simulink model "cuurent_controlled_circuit"  (R2022a)
settings: Solver=VariableStepAuto  StartTime=0.0  StopTime=25.0  RelTol=1e-3
undefined symbols (not defined in the file or in its folder): DiscIntNeverNeededParam
libraries: fl_lib x82, nesl_utility x65, eeRmsMeasurement x34, eePowerMeasurement x17, ee_lib x16
(part 2 of 3)

== system cuurent_controlled_circuit/Subsystem2 ==
  Display3 : Display
  Display4 : Display
  Display5 : Display
  PS-Simulink Converter2 : nesl_utility/PS-Simulink Converter  PhysicalDomain=network_engine_domain  SubClassName=ps_output  LeftPortType=input  RightPortType=output  PseudoPeriodic=off  Frequencies=[]  VectorFormat=inherit  Unit=inherit  AffineConversion=off
      settings: SourceProductBaseCode=SS,PW,VE
  PS-Simulink Converter3 : nesl_utility/PS-Simulink Converter  PhysicalDomain=network_engine_domain  SubClassName=ps_output  LeftPortType=input  RightPortType=output  PseudoPeriodic=off  Frequencies=[]  VectorFormat=inherit  Unit=inherit  AffineConversion=off
      settings: SourceProductBaseCode=SS,PW,VE
  Power Measurement2 : eePowerMeasurement/Power Measurement  LabelModeActiveChoice=Continuous  F=50  K=[0 1 2 3]  Ts=0
      settings: SourceProductBaseCode=PS
  RMS Measurement2 : eeRmsMeasurement/RMS Measurement  LabelModeActiveChoice=Total  F=50  SpecifyHarmonics=off  K=[0 1 2]  Ts=0
      settings: SourceProductBaseCode=PS
  RMS Measurement3 : eeRmsMeasurement/RMS Measurement  LabelModeActiveChoice=Total  F=50  SpecifyHarmonics=off  K=[0 1 2]  Ts=0
      settings: SourceProductBaseCode=PS
  Scope{6..10} (5 alike) : Scope
  input : PMIOPort  Side=Left
  input1 : PMIOPort  Port=2  Side=Left
  Q : Outport
  wires:
  Power Measurement2/2 -> Q/1
  PS-Simulink Converter3/1 -> RMS Measurement3/1, Scope8/1
  Power Measurement2/1 -> Display5/1, Scope10/1
  RMS Measurement2/1 -> Scope7/1, Display3/1, Power Measurement2/1
  PS-Simulink Converter2/1 -> RMS Measurement2/1, Scope6/1
  RMS Measurement3/1 -> Power Measurement2/2, Scope9/1, Display4/1
  connections:
  PS-Simulink Converter3/LConn1 -- input1/RConn1
  PS-Simulink Converter2/LConn1 -- input/RConn1

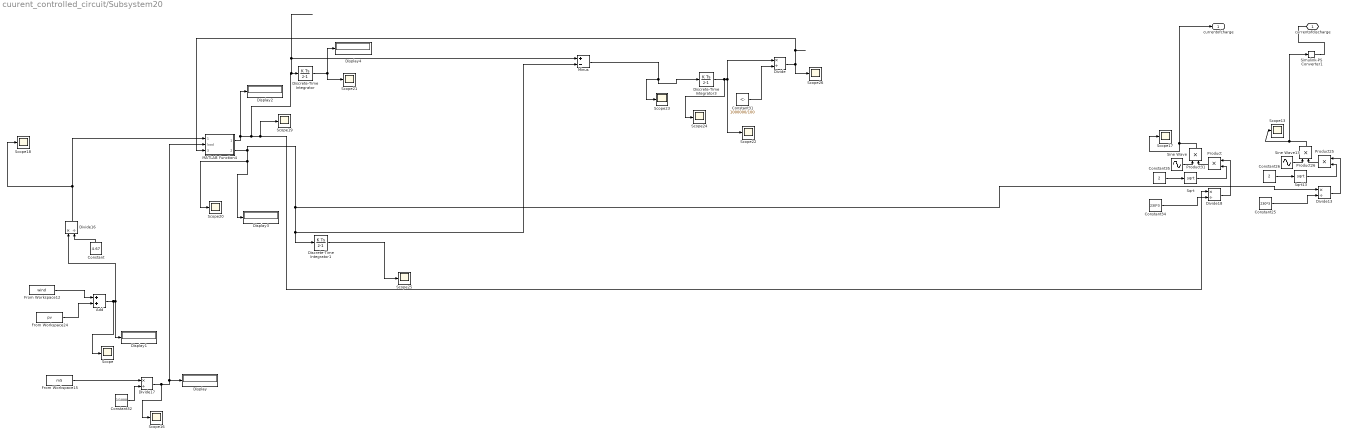
== system cuurent_controlled_circuit/Subsystem20 ==
  Add : Sum
  Constant : Constant  Value=4.67
  Constant25 : Constant  Value=230*3
  Constant26 : Constant  Value=2
  Constant31 : Constant  Value=1000000/100
  Constant32 : Constant  Value=1/1000
  Constant34 : Constant  Value=230*3
  Constant35 : Constant  Value=2
  Discrete-Time Integrator : DiscreteIntegrator  ICPrevOutput=DiscIntNeverNeededParam  ICPrevScaledInput=DiscIntNeverNeededParam
  Discrete-Time Integrator1 : DiscreteIntegrator  ICPrevOutput=DiscIntNeverNeededParam  ICPrevScaledInput=DiscIntNeverNeededParam
  Discrete-Time Integrator3 : DiscreteIntegrator  InitialCondition=500000  ICPrevOutput=DiscIntNeverNeededParam  ICPrevScaledInput=DiscIntNeverNeededParam
  Display{,1..4} (5 alike) : Display
  Divide{,13,16..18} (5 alike) : Product  Inputs=*/
  From Workspace12 : FromWorkspace  VariableName=wind  SampleTime=1  Interpolate=off  OutputAfterFinalValue=Holding final value
  From Workspace15 : FromWorkspace  VariableName=m5  SampleTime=1  Interpolate=off  OutputAfterFinalValue=Holding final value
  From Workspace24 : FromWorkspace  VariableName=pv  SampleTime=1  Interpolate=off  OutputAfterFinalValue=Holding final value
  MATLAB Function4 : MATLAB Function  TreatAsAtomicUnit=on
  Minus : Sum  Inputs=+-
  Product{,25..26,31} (4 alike) : Product
  Scope{,13,16..26} (13 alike) : Scope
  Simulink-PS Converter1 : nesl_utility/Simulink-PS Converter  PhysicalDomain=network_engine_domain  SubClassName=ps_input  LeftPortType=input  RightPortType=output  PseudoPeriodic=off  Frequencies=[]  NoiseDistribution=none  NoiseParameters=[]  Unit=1  AffineConversion=off  FilteringAndDerivatives=provide  SimscapeFilterOrder=1  InputFilterTimeConstant=0.001  UdotUserProvided=0
      settings: SourceProductBaseCode=SS,PW,VE
  Sine Wave : Sin  TimeSource=Use external signal  Frequency=314.6  Phase=240  SampleTime=0
  Sine Wave13 : Sin  Frequency=314.6  Phase=240  SampleTime=0
  Sqrt : Sqrt
  Sqrt13 : Sqrt
  currentofdischarge : PMIOPort  Side=Right
  currentofcharge : Outport
  wires:
  MATLAB Function4/1(charge) -> Minus/1, Discrete-Time Integrator/1, Divide18/1, Scope19/1, Display2/1
  MATLAB Function4/2(discharge) -> Divide13/1, Minus/2, Discrete-Time Integrator1/1, Scope20/1, Display3/1
  Divide/1 -> MATLAB Function4/3(batterycharge), Scope26/1
  Sine Wave13/1 -> Product26/1
  Product26/1 -> Simulink-PS Converter1/1, Scope13/1
  Discrete-Time Integrator/1 -> Display4/1, Scope21/1
  From Workspace24/1 -> Add/2
  Constant35/1 -> Sqrt/1
  Constant26/1 -> Sqrt13/1
  Product31/1 -> currentofcharge/1, Scope17/1
  Divide17/1 -> Scope16/1, MATLAB Function4/2(load), Display/1
  Divide13/1 -> Product25/1
  Add/1 -> Scope/1, Divide16/1, Display1/1
  Constant31/1 -> Divide/2
  Discrete-Time Integrator1/1 -> Scope25/1
  From Workspace15/1 -> Divide17/1
  Constant32/1 -> Divide17/2
  Minus/1 -> Discrete-Time Integrator3/1, Scope23/1
  Divide18/1 -> Product/1
  Discrete-Time Integrator3/1 -> Scope24/1, Divide/1, Scope22/1
  Product/1 -> Product31/2
  Product25/1 -> Product26/2
  Constant25/1 -> Divide13/2
  Constant/1 -> Divide16/2
  Divide16/1 -> Scope18/1, MATLAB Function4/1(pvandwind)
  Sine Wave/1 -> Product31/1
  Constant34/1 -> Divide18/2
  Sqrt/1 -> Product/2
  Sqrt13/1 -> Product25/2
  From Workspace12/1 -> Add/1
  connections:
  Simulink-PS Converter1/RConn1 -- currentofdischarge/RConn1

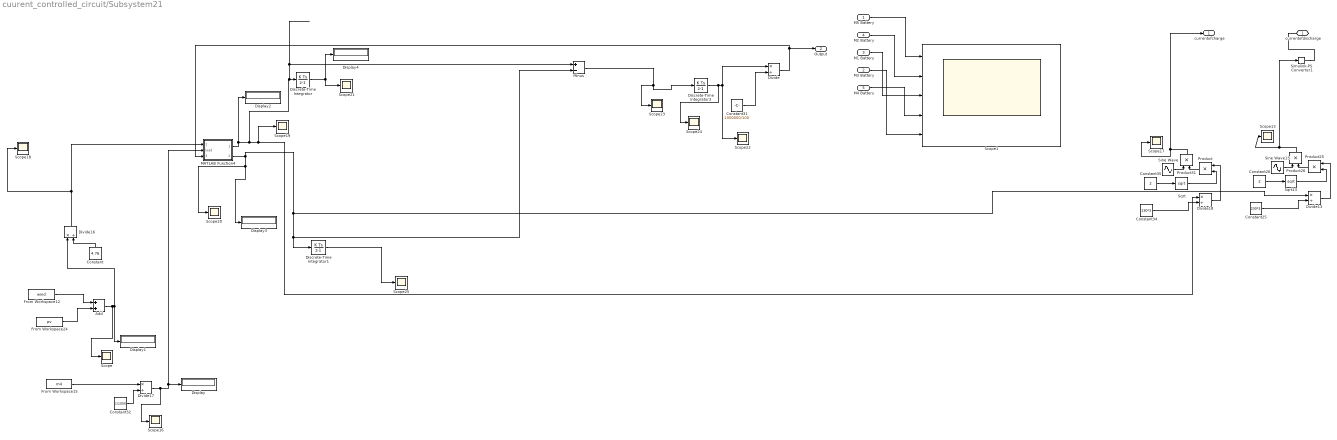
== system cuurent_controlled_circuit/Subsystem21 ==
  M5 Battery : Inport
  M3 Battery : Inport  Port=2
  M1 Battery : Inport  Port=3
  M2 Battery : Inport  Port=4
  M4 Battery : Inport  Port=5
  Add : Sum
  Constant : Constant  Value=4.76
  Constant25 : Constant  Value=230*3
  Constant26 : Constant  Value=2
  Constant31 : Constant  Value=1000000/100
  Constant32 : Constant  Value=1/1000
  Constant34 : Constant  Value=230*3
  Constant35 : Constant  Value=2
  Discrete-Time Integrator : DiscreteIntegrator  ICPrevOutput=DiscIntNeverNeededParam  ICPrevScaledInput=DiscIntNeverNeededParam
  Discrete-Time Integrator1 : DiscreteIntegrator  ICPrevOutput=DiscIntNeverNeededParam  ICPrevScaledInput=DiscIntNeverNeededParam
  Discrete-Time Integrator3 : DiscreteIntegrator  InitialCondition=500000  ICPrevOutput=DiscIntNeverNeededParam  ICPrevScaledInput=DiscIntNeverNeededParam
  Display{,1..4} (5 alike) : Display
  Divide{,13,16..18} (5 alike) : Product  Inputs=*/
  From Workspace12 : FromWorkspace  VariableName=wind  SampleTime=1  Interpolate=off  OutputAfterFinalValue=Holding final value
  From Workspace15 : FromWorkspace  VariableName=m4  SampleTime=1  Interpolate=off  OutputAfterFinalValue=Holding final value
  From Workspace24 : FromWorkspace  VariableName=pv  SampleTime=1  Interpolate=off  OutputAfterFinalValue=Holding final value
  MATLAB Function4 : MATLAB Function  TreatAsAtomicUnit=on
  Minus : Sum  Inputs=+-
  Product{,25..26,31} (4 alike) : Product
  Scope{,13,16..25} (12 alike) : Scope
  Scope1 : Scope  NumInputPorts=5
  Simulink-PS Converter1 : nesl_utility/Simulink-PS Converter  PhysicalDomain=network_engine_domain  SubClassName=ps_input  LeftPortType=input  RightPortType=output  PseudoPeriodic=off  Frequencies=[]  NoiseDistribution=none  NoiseParameters=[]  Unit=1  AffineConversion=off  FilteringAndDerivatives=provide  SimscapeFilterOrder=1  InputFilterTimeConstant=0.001  UdotUserProvided=0
      settings: SourceProductBaseCode=SS,PW,VE
  Sine Wave : Sin  Frequency=314.6  SampleTime=0
  Sine Wave13 : Sin  Frequency=314.6  SampleTime=0
  Sqrt : Sqrt
  Sqrt13 : Sqrt
  currentofdischarge : PMIOPort  Side=Right
  currentofcharge : Outport
  Output : Outport  Port=2
  wires:
  MATLAB Function4/1(charge) -> Minus/1, Discrete-Time Integrator/1, Divide18/1, Scope19/1, Display2/1
  MATLAB Function4/2(discharge) -> Divide13/1, Minus/2, Discrete-Time Integrator1/1, Scope20/1, Display3/1
  Sine Wave13/1 -> Product26/1
  Product26/1 -> Simulink-PS Converter1/1, Scope13/1
  Discrete-Time Integrator/1 -> Display4/1, Scope21/1
  From Workspace24/1 -> Add/2
  Constant35/1 -> Sqrt/1
  Constant26/1 -> Sqrt13/1
  Product31/1 -> currentofcharge/1, Scope17/1
  Divide17/1 -> Scope16/1, MATLAB Function4/2(load), Display/1
  Divide13/1 -> Product25/1
  Add/1 -> Scope/1, Divide16/1, Display1/1
  Constant31/1 -> Divide/2
  Discrete-Time Integrator1/1 -> Scope25/1
  From Workspace15/1 -> Divide17/1
  Constant32/1 -> Divide17/2
  Minus/1 -> Discrete-Time Integrator3/1, Scope23/1
  Divide18/1 -> Product/1
  Discrete-Time Integrator3/1 -> Scope24/1, Divide/1, Scope22/1
  Product/1 -> Product31/2
  Product25/1 -> Product26/2
  Constant25/1 -> Divide13/2
  Constant/1 -> Divide16/2
  Divide16/1 -> Scope18/1, MATLAB Function4/1(pvandwind)
  Sine Wave/1 -> Product31/1
  Constant34/1 -> Divide18/2
  Sqrt/1 -> Product/2
  Sqrt13/1 -> Product25/2
  From Workspace12/1 -> Add/1
  M5 Battery/1 -> Scope1/1
  M2 Battery/1 -> Scope1/2
  M1 Battery/1 -> Scope1/3
  M3 Battery/1 -> Scope1/5
  Divide/1 -> Output/1, MATLAB Function4/3(batterycharge)
  M4 Battery/1 -> Scope1/4
  connections:
  Simulink-PS Converter1/RConn1 -- currentofdischarge/RConn1

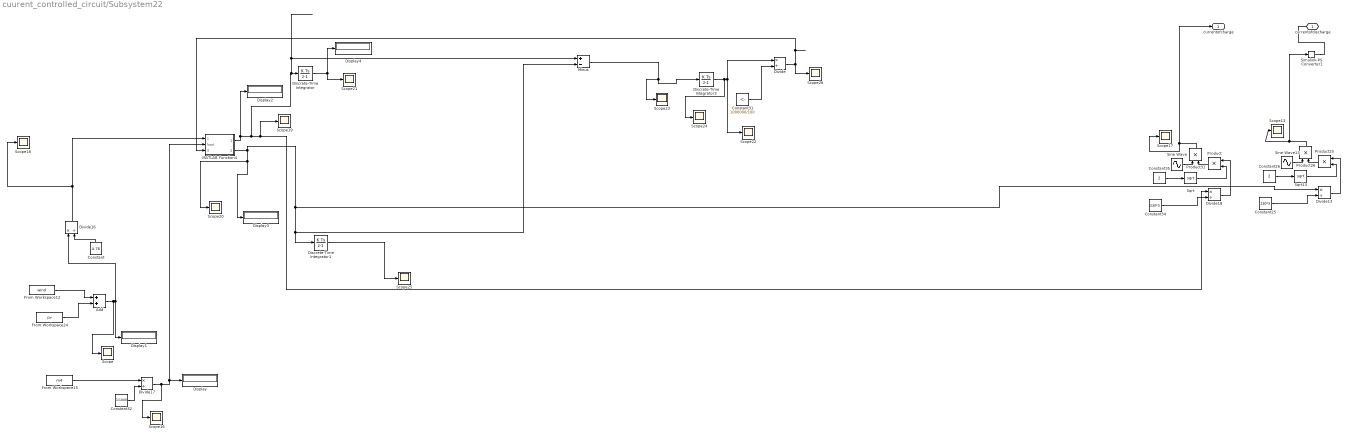
== system cuurent_controlled_circuit/Subsystem22 ==
  Add : Sum
  Constant : Constant  Value=4.76
  Constant25 : Constant  Value=230*3
  Constant26 : Constant  Value=2
  Constant31 : Constant  Value=1000000/100
  Constant32 : Constant  Value=1/1000
  Constant34 : Constant  Value=230*3
  Constant35 : Constant  Value=2
  Discrete-Time Integrator : DiscreteIntegrator  ICPrevOutput=DiscIntNeverNeededParam  ICPrevScaledInput=DiscIntNeverNeededParam
  Discrete-Time Integrator1 : DiscreteIntegrator  ICPrevOutput=DiscIntNeverNeededParam  ICPrevScaledInput=DiscIntNeverNeededParam
  Discrete-Time Integrator3 : DiscreteIntegrator  InitialCondition=500000  ICPrevOutput=DiscIntNeverNeededParam  ICPrevScaledInput=DiscIntNeverNeededParam
  Display{,1..4} (5 alike) : Display
  Divide{,13,16..18} (5 alike) : Product  Inputs=*/
  From Workspace12 : FromWorkspace  VariableName=wind  SampleTime=1  Interpolate=off  OutputAfterFinalValue=Holding final value
  From Workspace15 : FromWorkspace  VariableName=m4  SampleTime=1  Interpolate=off  OutputAfterFinalValue=Holding final value
  From Workspace24 : FromWorkspace  VariableName=pv  SampleTime=1  Interpolate=off  OutputAfterFinalValue=Holding final value
  MATLAB Function4 : MATLAB Function  TreatAsAtomicUnit=on
  Minus : Sum  Inputs=+-
  Product{,25..26,31} (4 alike) : Product
  Scope{,13,16..26} (13 alike) : Scope
  Simulink-PS Converter1 : nesl_utility/Simulink-PS Converter  PhysicalDomain=network_engine_domain  SubClassName=ps_input  LeftPortType=input  RightPortType=output  PseudoPeriodic=off  Frequencies=[]  NoiseDistribution=none  NoiseParameters=[]  Unit=1  AffineConversion=off  FilteringAndDerivatives=provide  SimscapeFilterOrder=1  InputFilterTimeConstant=0.001  UdotUserProvided=0
      settings: SourceProductBaseCode=SS,PW,VE
  Sine Wave : Sin  Frequency=314.6  Phase=120  SampleTime=0
  Sine Wave13 : Sin  Frequency=314.6  Phase=120  SampleTime=0
  Sqrt : Sqrt
  Sqrt13 : Sqrt
  currentofdischarge : PMIOPort  Side=Right
  currentofcharge : Outport
  wires:
  MATLAB Function4/1(charge) -> Minus/1, Discrete-Time Integrator/1, Divide18/1, Scope19/1, Display2/1
  MATLAB Function4/2(discharge) -> Divide13/1, Minus/2, Discrete-Time Integrator1/1, Scope20/1, Display3/1
  Divide/1 -> MATLAB Function4/3(batterycharge), Scope26/1
  Sine Wave13/1 -> Product26/1
  Product26/1 -> Simulink-PS Converter1/1, Scope13/1
  Discrete-Time Integrator/1 -> Display4/1, Scope21/1
  From Workspace24/1 -> Add/2
  Constant35/1 -> Sqrt/1
  Constant26/1 -> Sqrt13/1
  Product31/1 -> currentofcharge/1, Scope17/1
  Divide17/1 -> Scope16/1, MATLAB Function4/2(load), Display/1
  Divide13/1 -> Product25/1
  Add/1 -> Scope/1, Divide16/1, Display1/1
  Constant31/1 -> Divide/2
  Discrete-Time Integrator1/1 -> Scope25/1
  From Workspace15/1 -> Divide17/1
  Constant32/1 -> Divide17/2
  Minus/1 -> Discrete-Time Integrator3/1, Scope23/1
  Divide18/1 -> Product/1
  Discrete-Time Integrator3/1 -> Scope24/1, Divide/1, Scope22/1
  Product/1 -> Product31/2
  Product25/1 -> Product26/2
  Constant25/1 -> Divide13/2
  Constant/1 -> Divide16/2
  Divide16/1 -> Scope18/1, MATLAB Function4/1(pvandwind)
  Sine Wave/1 -> Product31/1
  Constant34/1 -> Divide18/2
  Sqrt/1 -> Product/2
  Sqrt13/1 -> Product25/2
  From Workspace12/1 -> Add/1
  connections:
  Simulink-PS Converter1/RConn1 -- currentofdischarge/RConn1

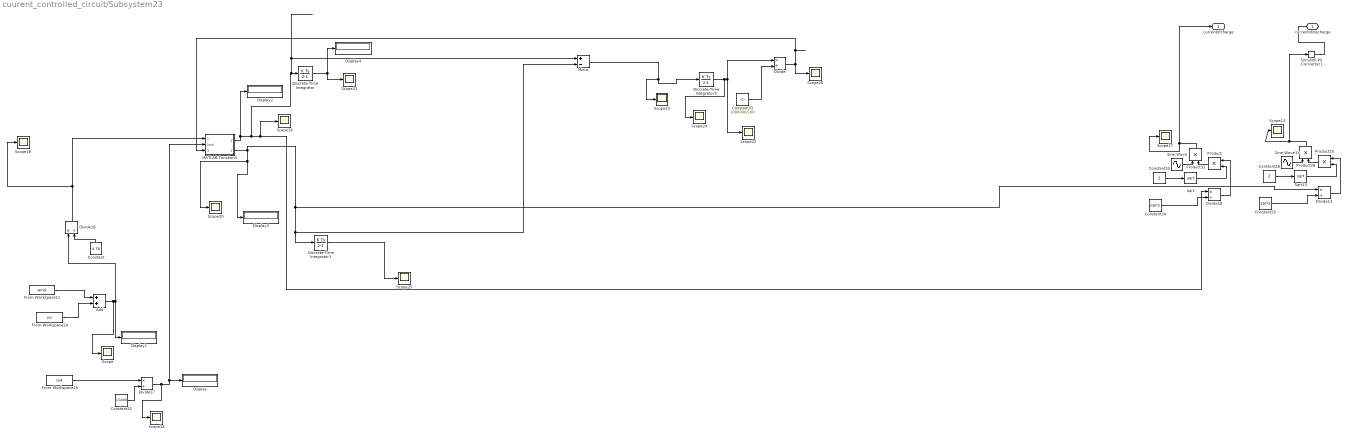
== system cuurent_controlled_circuit/Subsystem23 ==
  Add : Sum
  Constant : Constant  Value=4.76
  Constant25 : Constant  Value=230*3
  Constant26 : Constant  Value=2
  Constant31 : Constant  Value=1000000/100
  Constant32 : Constant  Value=1/1000
  Constant34 : Constant  Value=230*3
  Constant35 : Constant  Value=2
  Discrete-Time Integrator : DiscreteIntegrator  ICPrevOutput=DiscIntNeverNeededParam  ICPrevScaledInput=DiscIntNeverNeededParam
  Discrete-Time Integrator1 : DiscreteIntegrator  ICPrevOutput=DiscIntNeverNeededParam  ICPrevScaledInput=DiscIntNeverNeededParam
  Discrete-Time Integrator3 : DiscreteIntegrator  InitialCondition=500000  ICPrevOutput=DiscIntNeverNeededParam  ICPrevScaledInput=DiscIntNeverNeededParam
  Display{,1..4} (5 alike) : Display
  Divide{,13,16..18} (5 alike) : Product  Inputs=*/
  From Workspace12 : FromWorkspace  VariableName=wind  SampleTime=1  Interpolate=off  OutputAfterFinalValue=Holding final value
  From Workspace15 : FromWorkspace  VariableName=m4  SampleTime=1  Interpolate=off  OutputAfterFinalValue=Holding final value
  From Workspace24 : FromWorkspace  VariableName=pv  SampleTime=1  Interpolate=off  OutputAfterFinalValue=Holding final value
  MATLAB Function4 : MATLAB Function  TreatAsAtomicUnit=on
  Minus : Sum  Inputs=+-
  Product{,25..26,31} (4 alike) : Product
  Scope{,13,16..26} (13 alike) : Scope
  Simulink-PS Converter1 : nesl_utility/Simulink-PS Converter  PhysicalDomain=network_engine_domain  SubClassName=ps_input  LeftPortType=input  RightPortType=output  PseudoPeriodic=off  Frequencies=[]  NoiseDistribution=none  NoiseParameters=[]  Unit=1  AffineConversion=off  FilteringAndDerivatives=provide  SimscapeFilterOrder=1  InputFilterTimeConstant=0.001  UdotUserProvided=0
      settings: SourceProductBaseCode=SS,PW,VE
  Sine Wave : Sin  Frequency=314.6  Phase=240  SampleTime=0
  Sine Wave13 : Sin  Frequency=314.6  Phase=240  SampleTime=0
  Sqrt : Sqrt
  Sqrt13 : Sqrt
  currentofdischarge : PMIOPort  Side=Right
  currentofcharge : Outport
  wires:
  MATLAB Function4/1(charge) -> Minus/1, Discrete-Time Integrator/1, Divide18/1, Scope19/1, Display2/1
  MATLAB Function4/2(discharge) -> Divide13/1, Minus/2, Discrete-Time Integrator1/1, Scope20/1, Display3/1
  Divide/1 -> MATLAB Function4/3(batterycharge), Scope26/1
  Sine Wave13/1 -> Product26/1
  Product26/1 -> Simulink-PS Converter1/1, Scope13/1
  Discrete-Time Integrator/1 -> Display4/1, Scope21/1
  From Workspace24/1 -> Add/2
  Constant35/1 -> Sqrt/1
  Constant26/1 -> Sqrt13/1
  Product31/1 -> currentofcharge/1, Scope17/1
  Divide17/1 -> Scope16/1, MATLAB Function4/2(load), Display/1
  Divide13/1 -> Product25/1
  Add/1 -> Scope/1, Divide16/1, Display1/1
  Constant31/1 -> Divide/2
  Discrete-Time Integrator1/1 -> Scope25/1
  From Workspace15/1 -> Divide17/1
  Constant32/1 -> Divide17/2
  Minus/1 -> Discrete-Time Integrator3/1, Scope23/1
  Divide18/1 -> Product/1
  Discrete-Time Integrator3/1 -> Scope24/1, Divide/1, Scope22/1
  Product/1 -> Product31/2
  Product25/1 -> Product26/2
  Constant25/1 -> Divide13/2
  Constant/1 -> Divide16/2
  Divide16/1 -> Scope18/1, MATLAB Function4/1(pvandwind)
  Sine Wave/1 -> Product31/1
  Constant34/1 -> Divide18/2
  Sqrt/1 -> Product/2
  Sqrt13/1 -> Product25/2
  From Workspace12/1 -> Add/1
  connections:
  Simulink-PS Converter1/RConn1 -- currentofdischarge/RConn1

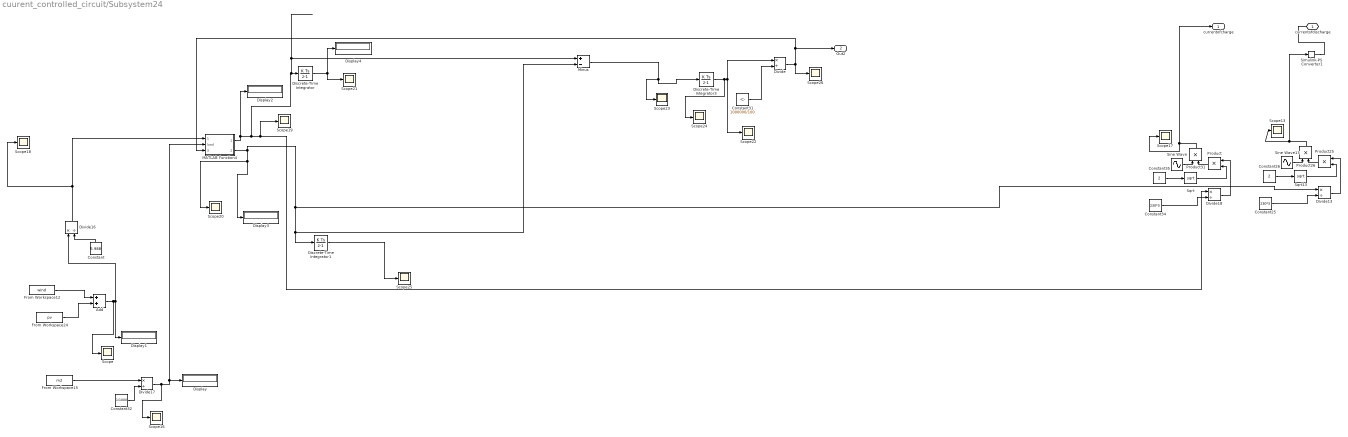
== system cuurent_controlled_circuit/Subsystem24 ==
  Add : Sum
  Constant : Constant  Value=5.988
  Constant25 : Constant  Value=230*3
  Constant26 : Constant  Value=2
  Constant31 : Constant  Value=1000000/100
  Constant32 : Constant  Value=1/1000
  Constant34 : Constant  Value=230*3
  Constant35 : Constant  Value=2
  Discrete-Time Integrator : DiscreteIntegrator  ICPrevOutput=DiscIntNeverNeededParam  ICPrevScaledInput=DiscIntNeverNeededParam
  Discrete-Time Integrator1 : DiscreteIntegrator  ICPrevOutput=DiscIntNeverNeededParam  ICPrevScaledInput=DiscIntNeverNeededParam
  Discrete-Time Integrator3 : DiscreteIntegrator  InitialCondition=500000  ICPrevOutput=DiscIntNeverNeededParam  ICPrevScaledInput=DiscIntNeverNeededParam
  Display{,1..4} (5 alike) : Display
  Divide{,13,16..18} (5 alike) : Product  Inputs=*/
  From Workspace12 : FromWorkspace  VariableName=wind  SampleTime=1  Interpolate=off  OutputAfterFinalValue=Holding final value
  From Workspace15 : FromWorkspace  VariableName=m2  SampleTime=1  Interpolate=off  OutputAfterFinalValue=Holding final value
  From Workspace24 : FromWorkspace  VariableName=pv  SampleTime=1  Interpolate=off  OutputAfterFinalValue=Holding final value
  MATLAB Function4 : MATLAB Function  TreatAsAtomicUnit=on
  Minus : Sum  Inputs=+-
  Product{,25..26,31} (4 alike) : Product
  Scope{,13,16..26} (13 alike) : Scope
  Simulink-PS Converter1 : nesl_utility/Simulink-PS Converter  PhysicalDomain=network_engine_domain  SubClassName=ps_input  LeftPortType=input  RightPortType=output  PseudoPeriodic=off  Frequencies=[]  NoiseDistribution=none  NoiseParameters=[]  Unit=1  AffineConversion=off  FilteringAndDerivatives=provide  SimscapeFilterOrder=1  InputFilterTimeConstant=0.001  UdotUserProvided=0
      settings: SourceProductBaseCode=SS,PW,VE
  Sine Wave : Sin  Frequency=314.6  SampleTime=0
  Sine Wave13 : Sin  Frequency=314.6  SampleTime=0
  Sqrt : Sqrt
  Sqrt13 : Sqrt
  currentofdischarge : PMIOPort  Side=Right
  currentofcharge : Outport
  Out2 : Outport  Port=2
  wires:
  MATLAB Function4/1(charge) -> Minus/1, Discrete-Time Integrator/1, Divide18/1, Scope19/1, Display2/1
  MATLAB Function4/2(discharge) -> Divide13/1, Minus/2, Discrete-Time Integrator1/1, Scope20/1, Display3/1
  Sine Wave13/1 -> Product26/1
  Product26/1 -> Simulink-PS Converter1/1, Scope13/1
  Discrete-Time Integrator/1 -> Display4/1, Scope21/1
  From Workspace24/1 -> Add/2
  Constant35/1 -> Sqrt/1
  Constant26/1 -> Sqrt13/1
  Product31/1 -> currentofcharge/1, Scope17/1
  Divide17/1 -> Scope16/1, MATLAB Function4/2(load), Display/1
  Divide13/1 -> Product25/1
  Add/1 -> Scope/1, Divide16/1, Display1/1
  Constant31/1 -> Divide/2
  Discrete-Time Integrator1/1 -> Scope25/1
  From Workspace15/1 -> Divide17/1
  Constant32/1 -> Divide17/2
  Minus/1 -> Discrete-Time Integrator3/1, Scope23/1
  Divide18/1 -> Product/1
  Discrete-Time Integrator3/1 -> Scope24/1, Divide/1, Scope22/1
  Product/1 -> Product31/2
  Product25/1 -> Product26/2
  Constant25/1 -> Divide13/2
  Constant/1 -> Divide16/2
  Divide16/1 -> Scope18/1, MATLAB Function4/1(pvandwind)
  Sine Wave/1 -> Product31/1
  Constant34/1 -> Divide18/2
  Sqrt/1 -> Product/2
  Sqrt13/1 -> Product25/2
  From Workspace12/1 -> Add/1
  Divide/1 -> Out2/1, MATLAB Function4/3(batterycharge), Scope26/1
  connections:
  Simulink-PS Converter1/RConn1 -- currentofdischarge/RConn1

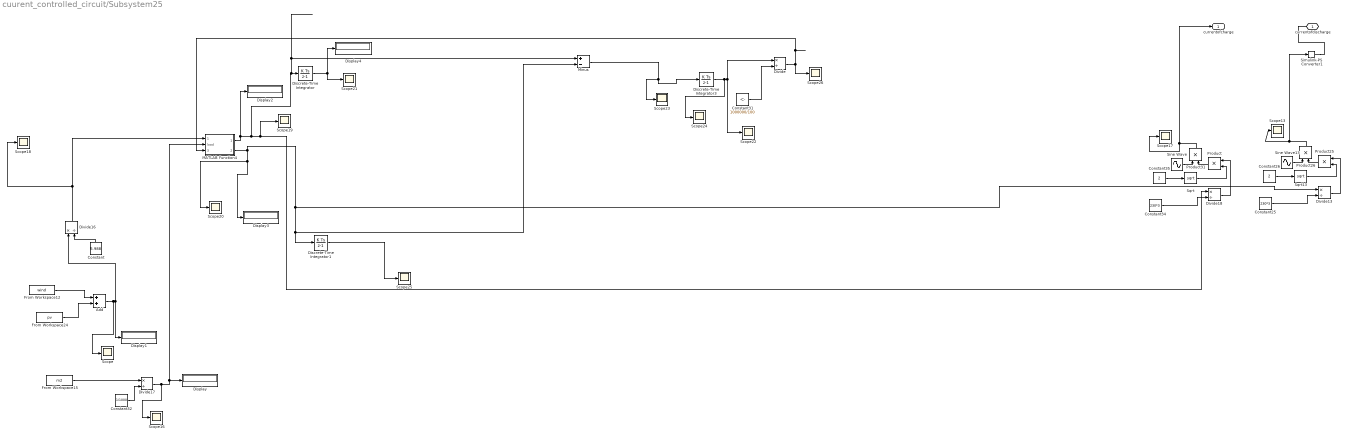
== system cuurent_controlled_circuit/Subsystem25 ==
  Add : Sum
  Constant : Constant  Value=5.988
  Constant25 : Constant  Value=230*3
  Constant26 : Constant  Value=2
  Constant31 : Constant  Value=1000000/100
  Constant32 : Constant  Value=1/1000
  Constant34 : Constant  Value=230*3
  Constant35 : Constant  Value=2
  Discrete-Time Integrator : DiscreteIntegrator  ICPrevOutput=DiscIntNeverNeededParam  ICPrevScaledInput=DiscIntNeverNeededParam
  Discrete-Time Integrator1 : DiscreteIntegrator  ICPrevOutput=DiscIntNeverNeededParam  ICPrevScaledInput=DiscIntNeverNeededParam
  Discrete-Time Integrator3 : DiscreteIntegrator  InitialCondition=500000  ICPrevOutput=DiscIntNeverNeededParam  ICPrevScaledInput=DiscIntNeverNeededParam
  Display{,1..4} (5 alike) : Display
  Divide{,13,16..18} (5 alike) : Product  Inputs=*/
  From Workspace12 : FromWorkspace  VariableName=wind  SampleTime=1  Interpolate=off  OutputAfterFinalValue=Holding final value
  From Workspace15 : FromWorkspace  VariableName=m2  SampleTime=1  Interpolate=off  OutputAfterFinalValue=Holding final value
  From Workspace24 : FromWorkspace  VariableName=pv  SampleTime=1  Interpolate=off  OutputAfterFinalValue=Holding final value
  MATLAB Function4 : MATLAB Function  TreatAsAtomicUnit=on
  Minus : Sum  Inputs=+-
  Product{,25..26,31} (4 alike) : Product
  Scope{,13,16..26} (13 alike) : Scope
  Simulink-PS Converter1 : nesl_utility/Simulink-PS Converter  PhysicalDomain=network_engine_domain  SubClassName=ps_input  LeftPortType=input  RightPortType=output  PseudoPeriodic=off  Frequencies=[]  NoiseDistribution=none  NoiseParameters=[]  Unit=1  AffineConversion=off  FilteringAndDerivatives=provide  SimscapeFilterOrder=1  InputFilterTimeConstant=0.001  UdotUserProvided=0
      settings: SourceProductBaseCode=SS,PW,VE
  Sine Wave : Sin  Frequency=314.6  Phase=120  SampleTime=0
  Sine Wave13 : Sin  Frequency=314.6  Phase=120  SampleTime=0
  Sqrt : Sqrt
  Sqrt13 : Sqrt
  currentofdischarge : PMIOPort  Side=Right
  currentofcharge : Outport
  wires:
  MATLAB Function4/1(charge) -> Minus/1, Discrete-Time Integrator/1, Divide18/1, Scope19/1, Display2/1
  MATLAB Function4/2(discharge) -> Divide13/1, Minus/2, Discrete-Time Integrator1/1, Scope20/1, Display3/1
  Divide/1 -> MATLAB Function4/3(batterycharge), Scope26/1
  Sine Wave13/1 -> Product26/1
  Product26/1 -> Simulink-PS Converter1/1, Scope13/1
  Discrete-Time Integrator/1 -> Display4/1, Scope21/1
  From Workspace24/1 -> Add/2
  Constant35/1 -> Sqrt/1
  Constant26/1 -> Sqrt13/1
  Product31/1 -> currentofcharge/1, Scope17/1
  Divide17/1 -> Scope16/1, MATLAB Function4/2(load), Display/1
  Divide13/1 -> Product25/1
  Add/1 -> Scope/1, Divide16/1, Display1/1
  Constant31/1 -> Divide/2
  Discrete-Time Integrator1/1 -> Scope25/1
  From Workspace15/1 -> Divide17/1
  Constant32/1 -> Divide17/2
  Minus/1 -> Discrete-Time Integrator3/1, Scope23/1
  Divide18/1 -> Product/1
  Discrete-Time Integrator3/1 -> Scope24/1, Divide/1, Scope22/1
  Product/1 -> Product31/2
  Product25/1 -> Product26/2
  Constant25/1 -> Divide13/2
  Constant/1 -> Divide16/2
  Divide16/1 -> Scope18/1, MATLAB Function4/1(pvandwind)
  Sine Wave/1 -> Product31/1
  Constant34/1 -> Divide18/2
  Sqrt/1 -> Product/2
  Sqrt13/1 -> Product25/2
  From Workspace12/1 -> Add/1
  connections:
  Simulink-PS Converter1/RConn1 -- currentofdischarge/RConn1

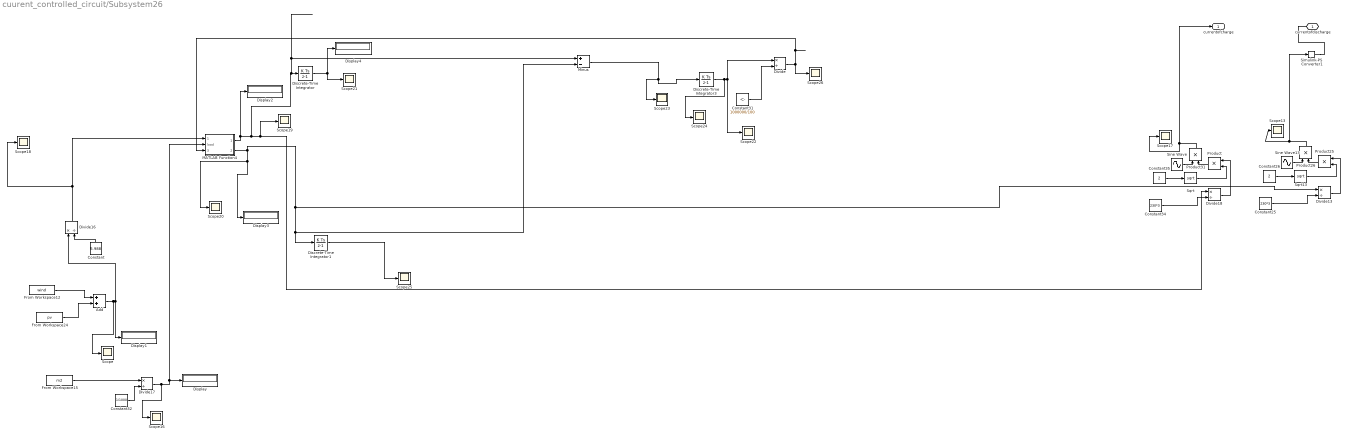
== system cuurent_controlled_circuit/Subsystem26 ==
  Add : Sum
  Constant : Constant  Value=5.988
  Constant25 : Constant  Value=230*3
  Constant26 : Constant  Value=2
  Constant31 : Constant  Value=1000000/100
  Constant32 : Constant  Value=1/1000
  Constant34 : Constant  Value=230*3
  Constant35 : Constant  Value=2
  Discrete-Time Integrator : DiscreteIntegrator  ICPrevOutput=DiscIntNeverNeededParam  ICPrevScaledInput=DiscIntNeverNeededParam
  Discrete-Time Integrator1 : DiscreteIntegrator  ICPrevOutput=DiscIntNeverNeededParam  ICPrevScaledInput=DiscIntNeverNeededParam
  Discrete-Time Integrator3 : DiscreteIntegrator  InitialCondition=500000  ICPrevOutput=DiscIntNeverNeededParam  ICPrevScaledInput=DiscIntNeverNeededParam
  Display{,1..4} (5 alike) : Display
  Divide{,13,16..18} (5 alike) : Product  Inputs=*/
  From Workspace12 : FromWorkspace  VariableName=wind  SampleTime=1  Interpolate=off  OutputAfterFinalValue=Holding final value
  From Workspace15 : FromWorkspace  VariableName=m2  SampleTime=1  Interpolate=off  OutputAfterFinalValue=Holding final value
  From Workspace24 : FromWorkspace  VariableName=pv  SampleTime=1  Interpolate=off  OutputAfterFinalValue=Holding final value
  MATLAB Function4 : MATLAB Function  TreatAsAtomicUnit=on
  Minus : Sum  Inputs=+-
  Product{,25..26,31} (4 alike) : Product
  Scope{,13,16..26} (13 alike) : Scope
  Simulink-PS Converter1 : nesl_utility/Simulink-PS Converter  PhysicalDomain=network_engine_domain  SubClassName=ps_input  LeftPortType=input  RightPortType=output  PseudoPeriodic=off  Frequencies=[]  NoiseDistribution=none  NoiseParameters=[]  Unit=1  AffineConversion=off  FilteringAndDerivatives=provide  SimscapeFilterOrder=1  InputFilterTimeConstant=0.001  UdotUserProvided=0
      settings: SourceProductBaseCode=SS,PW,VE
  Sine Wave : Sin  Frequency=314.6  Phase=240  SampleTime=0
  Sine Wave13 : Sin  Frequency=314.6  Phase=240  SampleTime=0
  Sqrt : Sqrt
  Sqrt13 : Sqrt
  currentofdischarge : PMIOPort  Side=Right
  currentofcharge : Outport
  wires:
  MATLAB Function4/1(charge) -> Minus/1, Discrete-Time Integrator/1, Divide18/1, Scope19/1, Display2/1
  MATLAB Function4/2(discharge) -> Divide13/1, Minus/2, Discrete-Time Integrator1/1, Scope20/1, Display3/1
  Divide/1 -> MATLAB Function4/3(batterycharge), Scope26/1
  Sine Wave13/1 -> Product26/1
  Product26/1 -> Simulink-PS Converter1/1, Scope13/1
  Discrete-Time Integrator/1 -> Display4/1, Scope21/1
  From Workspace24/1 -> Add/2
  Constant35/1 -> Sqrt/1
  Constant26/1 -> Sqrt13/1
  Product31/1 -> currentofcharge/1, Scope17/1
  Divide17/1 -> Scope16/1, MATLAB Function4/2(load), Display/1
  Divide13/1 -> Product25/1
  Add/1 -> Scope/1, Divide16/1, Display1/1
  Constant31/1 -> Divide/2
  Discrete-Time Integrator1/1 -> Scope25/1
  From Workspace15/1 -> Divide17/1
  Constant32/1 -> Divide17/2
  Minus/1 -> Discrete-Time Integrator3/1, Scope23/1
  Divide18/1 -> Product/1
  Discrete-Time Integrator3/1 -> Scope24/1, Divide/1, Scope22/1
  Product/1 -> Product31/2
  Product25/1 -> Product26/2
  Constant25/1 -> Divide13/2
  Constant/1 -> Divide16/2
  Divide16/1 -> Scope18/1, MATLAB Function4/1(pvandwind)
  Sine Wave/1 -> Product31/1
  Constant34/1 -> Divide18/2
  Sqrt/1 -> Product/2
  Sqrt13/1 -> Product25/2
  From Workspace12/1 -> Add/1
  connections:
  Simulink-PS Converter1/RConn1 -- currentofdischarge/RConn1

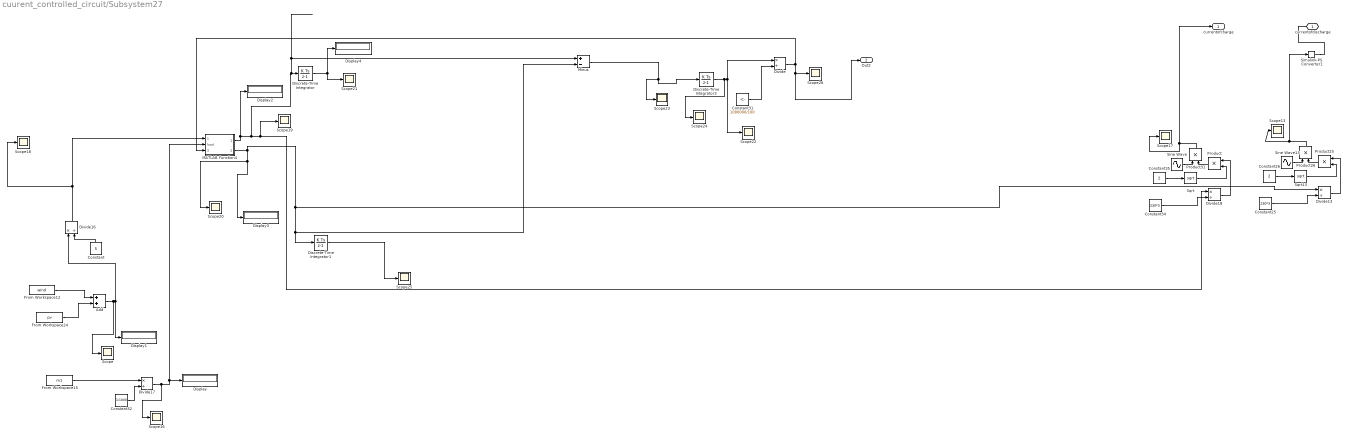
== system cuurent_controlled_circuit/Subsystem27 ==
  Add : Sum
  Constant : Constant  Value=5
  Constant25 : Constant  Value=230*3
  Constant26 : Constant  Value=2
  Constant31 : Constant  Value=1000000/100
  Constant32 : Constant  Value=1/1000
  Constant34 : Constant  Value=230*3
  Constant35 : Constant  Value=2
  Discrete-Time Integrator : DiscreteIntegrator  ICPrevOutput=DiscIntNeverNeededParam  ICPrevScaledInput=DiscIntNeverNeededParam
  Discrete-Time Integrator1 : DiscreteIntegrator  ICPrevOutput=DiscIntNeverNeededParam  ICPrevScaledInput=DiscIntNeverNeededParam
  Discrete-Time Integrator3 : DiscreteIntegrator  InitialCondition=500000  ICPrevOutput=DiscIntNeverNeededParam  ICPrevScaledInput=DiscIntNeverNeededParam
  Display{,1..4} (5 alike) : Display
  Divide{,13,16..18} (5 alike) : Product  Inputs=*/
  From Workspace12 : FromWorkspace  VariableName=wind  SampleTime=1  Interpolate=off  OutputAfterFinalValue=Holding final value
  From Workspace15 : FromWorkspace  VariableName=m1  SampleTime=1  Interpolate=off  OutputAfterFinalValue=Holding final value
  From Workspace24 : FromWorkspace  VariableName=pv  SampleTime=1  Interpolate=off  OutputAfterFinalValue=Holding final value
  MATLAB Function4 : MATLAB Function  TreatAsAtomicUnit=on
  Minus : Sum  Inputs=+-
  Product{,25..26,31} (4 alike) : Product
  Scope{,13,16..26} (13 alike) : Scope
  Simulink-PS Converter1 : nesl_utility/Simulink-PS Converter  PhysicalDomain=network_engine_domain  SubClassName=ps_input  LeftPortType=input  RightPortType=output  PseudoPeriodic=off  Frequencies=[]  NoiseDistribution=none  NoiseParameters=[]  Unit=1  AffineConversion=off  FilteringAndDerivatives=provide  SimscapeFilterOrder=1  InputFilterTimeConstant=0.001  UdotUserProvided=0
      settings: SourceProductBaseCode=SS,PW,VE
  Sine Wave : Sin  Frequency=314.6  SampleTime=0
  Sine Wave13 : Sin  Frequency=314.6  SampleTime=0
  Sqrt : Sqrt
  Sqrt13 : Sqrt
  currentofdischarge : PMIOPort  Side=Right
  currentofcharge : Outport
  Out2 : Outport  Port=2
  wires:
  MATLAB Function4/1(charge) -> Minus/1, Discrete-Time Integrator/1, Divide18/1, Scope19/1, Display2/1
  MATLAB Function4/2(discharge) -> Divide13/1, Minus/2, Discrete-Time Integrator1/1, Scope20/1, Display3/1
  Sine Wave13/1 -> Product26/1
  Product26/1 -> Simulink-PS Converter1/1, Scope13/1
  Discrete-Time Integrator/1 -> Display4/1, Scope21/1
  From Workspace24/1 -> Add/2
  Constant35/1 -> Sqrt/1
  Constant26/1 -> Sqrt13/1
  Product31/1 -> currentofcharge/1, Scope17/1
  Divide17/1 -> Scope16/1, MATLAB Function4/2(load), Display/1
  Divide13/1 -> Product25/1
  Add/1 -> Scope/1, Divide16/1, Display1/1
  Constant31/1 -> Divide/2
  Discrete-Time Integrator1/1 -> Scope25/1
  From Workspace15/1 -> Divide17/1
  Constant32/1 -> Divide17/2
  Minus/1 -> Discrete-Time Integrator3/1, Scope23/1
  Divide18/1 -> Product/1
  Discrete-Time Integrator3/1 -> Scope24/1, Divide/1, Scope22/1
  Product/1 -> Product31/2
  Product25/1 -> Product26/2
  Constant25/1 -> Divide13/2
  Constant/1 -> Divide16/2
  Divide16/1 -> Scope18/1, MATLAB Function4/1(pvandwind)
  Sine Wave/1 -> Product31/1
  Constant34/1 -> Divide18/2
  Sqrt/1 -> Product/2
  Sqrt13/1 -> Product25/2
  From Workspace12/1 -> Add/1
  Divide/1 -> Out2/1, Scope26/1, MATLAB Function4/3(batterycharge)
  connections:
  Simulink-PS Converter1/RConn1 -- currentofdischarge/RConn1

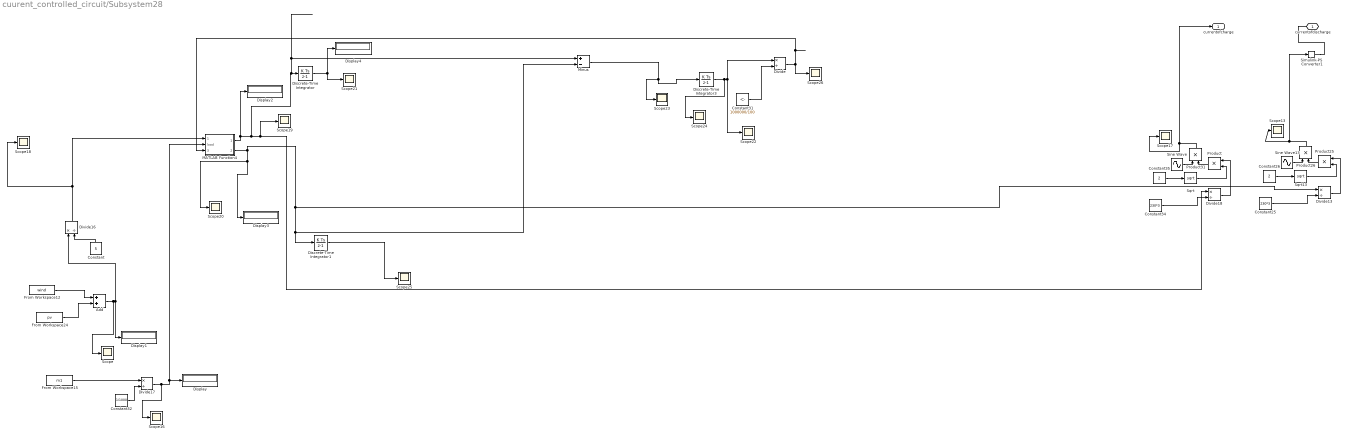
== system cuurent_controlled_circuit/Subsystem28 ==
  Add : Sum
  Constant : Constant  Value=5
  Constant25 : Constant  Value=230*3
  Constant26 : Constant  Value=2
  Constant31 : Constant  Value=1000000/100
  Constant32 : Constant  Value=1/1000
  Constant34 : Constant  Value=230*3
  Constant35 : Constant  Value=2
  Discrete-Time Integrator : DiscreteIntegrator  ICPrevOutput=DiscIntNeverNeededParam  ICPrevScaledInput=DiscIntNeverNeededParam
  Discrete-Time Integrator1 : DiscreteIntegrator  ICPrevOutput=DiscIntNeverNeededParam  ICPrevScaledInput=DiscIntNeverNeededParam
  Discrete-Time Integrator3 : DiscreteIntegrator  InitialCondition=500000  ICPrevOutput=DiscIntNeverNeededParam  ICPrevScaledInput=DiscIntNeverNeededParam
  Display{,1..4} (5 alike) : Display
  Divide{,13,16..18} (5 alike) : Product  Inputs=*/
  From Workspace12 : FromWorkspace  VariableName=wind  SampleTime=1  Interpolate=off  OutputAfterFinalValue=Holding final value
  From Workspace15 : FromWorkspace  VariableName=m1  SampleTime=1  Interpolate=off  OutputAfterFinalValue=Holding final value
  From Workspace24 : FromWorkspace  VariableName=pv  SampleTime=1  Interpolate=off  OutputAfterFinalValue=Holding final value
  MATLAB Function4 : MATLAB Function  TreatAsAtomicUnit=on
  Minus : Sum  Inputs=+-
  Product{,25..26,31} (4 alike) : Product
  Scope{,13,16..26} (13 alike) : Scope
  Simulink-PS Converter1 : nesl_utility/Simulink-PS Converter  PhysicalDomain=network_engine_domain  SubClassName=ps_input  LeftPortType=input  RightPortType=output  PseudoPeriodic=off  Frequencies=[]  NoiseDistribution=none  NoiseParameters=[]  Unit=1  AffineConversion=off  FilteringAndDerivatives=provide  SimscapeFilterOrder=1  InputFilterTimeConstant=0.001  UdotUserProvided=0
      settings: SourceProductBaseCode=SS,PW,VE
  Sine Wave : Sin  Frequency=314.6  Phase=120  SampleTime=0
  Sine Wave13 : Sin  Frequency=314.6  Phase=120  SampleTime=0
  Sqrt : Sqrt
  Sqrt13 : Sqrt
  currentofdischarge : PMIOPort  Side=Right
  currentofcharge : Outport
  wires:
  MATLAB Function4/1(charge) -> Minus/1, Discrete-Time Integrator/1, Divide18/1, Scope19/1, Display2/1
  MATLAB Function4/2(discharge) -> Divide13/1, Minus/2, Discrete-Time Integrator1/1, Scope20/1, Display3/1
  Divide/1 -> MATLAB Function4/3(batterycharge), Scope26/1
  Sine Wave13/1 -> Product26/1
  Product26/1 -> Simulink-PS Converter1/1, Scope13/1
  Discrete-Time Integrator/1 -> Display4/1, Scope21/1
  From Workspace24/1 -> Add/2
  Constant35/1 -> Sqrt/1
  Constant26/1 -> Sqrt13/1
  Product31/1 -> currentofcharge/1, Scope17/1
  Divide17/1 -> Scope16/1, MATLAB Function4/2(load), Display/1
  Divide13/1 -> Product25/1
  Add/1 -> Scope/1, Divide16/1, Display1/1
  Constant31/1 -> Divide/2
  Discrete-Time Integrator1/1 -> Scope25/1
  From Workspace15/1 -> Divide17/1
  Constant32/1 -> Divide17/2
  Minus/1 -> Discrete-Time Integrator3/1, Scope23/1
  Divide18/1 -> Product/1
  Discrete-Time Integrator3/1 -> Scope24/1, Divide/1, Scope22/1
  Product/1 -> Product31/2
  Product25/1 -> Product26/2
  Constant25/1 -> Divide13/2
  Constant/1 -> Divide16/2
  Divide16/1 -> Scope18/1, MATLAB Function4/1(pvandwind)
  Sine Wave/1 -> Product31/1
  Constant34/1 -> Divide18/2
  Sqrt/1 -> Product/2
  Sqrt13/1 -> Product25/2
  From Workspace12/1 -> Add/1
  connections:
  Simulink-PS Converter1/RConn1 -- currentofdischarge/RConn1

== system cuurent_controlled_circuit/Subsystem29 ==
  Add : Sum
  Constant : Constant  Value=5
  Constant25 : Constant  Value=230*3
  Constant26 : Constant  Value=2
  Constant31 : Constant  Value=1000000/100
  Constant32 : Constant  Value=1/1000
  Constant34 : Constant  Value=230*3
  Constant35 : Constant  Value=2
  Discrete-Time Integrator : DiscreteIntegrator  ICPrevOutput=DiscIntNeverNeededParam  ICPrevScaledInput=DiscIntNeverNeededParam
  Discrete-Time Integrator1 : DiscreteIntegrator  ICPrevOutput=DiscIntNeverNeededParam  ICPrevScaledInput=DiscIntNeverNeededParam
  Discrete-Time Integrator3 : DiscreteIntegrator  InitialCondition=500000  ICPrevOutput=DiscIntNeverNeededParam  ICPrevScaledInput=DiscIntNeverNeededParam
  Display{,1..4} (5 alike) : Display
  Divide{,13,16..18} (5 alike) : Product  Inputs=*/
  From Workspace12 : FromWorkspace  VariableName=wind  SampleTime=1  Interpolate=off  OutputAfterFinalValue=Holding final value
  From Workspace15 : FromWorkspace  VariableName=m1  SampleTime=1  Interpolate=off  OutputAfterFinalValue=Holding final value
  From Workspace24 : FromWorkspace  VariableName=pv  SampleTime=1  Interpolate=off  OutputAfterFinalValue=Holding final value
  MATLAB Function4 : MATLAB Function  TreatAsAtomicUnit=on
  Minus : Sum  Inputs=+-
  Product{,25..26,31} (4 alike) : Product
  Scope{,13,16..26} (13 alike) : Scope
  Simulink-PS Converter1 : nesl_utility/Simulink-PS Converter  PhysicalDomain=network_engine_domain  SubClassName=ps_input  LeftPortType=input  RightPortType=output  PseudoPeriodic=off  Frequencies=[]  NoiseDistribution=none  NoiseParameters=[]  Unit=1  AffineConversion=off  FilteringAndDerivatives=provide  SimscapeFilterOrder=1  InputFilterTimeConstant=0.001  UdotUserProvided=0
      settings: SourceProductBaseCode=SS,PW,VE
  Sine Wave : Sin  Frequency=314.6  Phase=240  SampleTime=0
  Sine Wave13 : Sin  Frequency=314.6  Phase=240  SampleTime=0
  Sqrt : Sqrt
  Sqrt13 : Sqrt
  currentofdischarge : PMIOPort  Side=Right
  currentofcharge : Outport
  wires:
  MATLAB Function4/1(charge) -> Minus/1, Discrete-Time Integrator/1, Divide18/1, Scope19/1, Display2/1
  MATLAB Function4/2(discharge) -> Divide13/1, Minus/2, Discrete-Time Integrator1/1, Scope20/1, Display3/1
  Divide/1 -> MATLAB Function4/3(batterycharge), Scope26/1
  Sine Wave13/1 -> Product26/1
  Product26/1 -> Simulink-PS Converter1/1, Scope13/1
  Discrete-Time Integrator/1 -> Display4/1, Scope21/1
  From Workspace24/1 -> Add/2
  Constant35/1 -> Sqrt/1
  Constant26/1 -> Sqrt13/1
  Product31/1 -> currentofcharge/1, Scope17/1
  Divide17/1 -> Scope16/1, MATLAB Function4/2(load), Display/1
  Divide13/1 -> Product25/1
  Add/1 -> Scope/1, Divide16/1, Display1/1
  Constant31/1 -> Divide/2
  Discrete-Time Integrator1/1 -> Scope25/1
  From Workspace15/1 -> Divide17/1
  Constant32/1 -> Divide17/2
  Minus/1 -> Discrete-Time Integrator3/1, Scope23/1
  Divide18/1 -> Product/1
  Discrete-Time Integrator3/1 -> Scope24/1, Divide/1, Scope22/1
  Product/1 -> Product31/2
  Product25/1 -> Product26/2
  Constant25/1 -> Divide13/2
  Constant/1 -> Divide16/2
  Divide16/1 -> Scope18/1, MATLAB Function4/1(pvandwind)
  Sine Wave/1 -> Product31/1
  Constant34/1 -> Divide18/2
  Sqrt/1 -> Product/2
  Sqrt13/1 -> Product25/2
  From Workspace12/1 -> Add/1
  connections:
  Simulink-PS Converter1/RConn1 -- currentofdischarge/RConn1

== system cuurent_controlled_circuit/Subsystem3 ==
  Display3 : Display
  Display4 : Display
  Display5 : Display
  PS-Simulink Converter2 : nesl_utility/PS-Simulink Converter  PhysicalDomain=network_engine_domain  SubClassName=ps_output  LeftPortType=input  RightPortType=output  PseudoPeriodic=off  Frequencies=[]  VectorFormat=inherit  Unit=inherit  AffineConversion=off
      settings: SourceProductBaseCode=SS,PW,VE
  PS-Simulink Converter3 : nesl_utility/PS-Simulink Converter  PhysicalDomain=network_engine_domain  SubClassName=ps_output  LeftPortType=input  RightPortType=output  PseudoPeriodic=off  Frequencies=[]  VectorFormat=inherit  Unit=inherit  AffineConversion=off
      settings: SourceProductBaseCode=SS,PW,VE
  Power Measurement2 : eePowerMeasurement/Power Measurement  LabelModeActiveChoice=Continuous  F=50  K=[0 1 2 3]  Ts=0
      settings: SourceProductBaseCode=PS
  RMS Measurement2 : eeRmsMeasurement/RMS Measurement  LabelModeActiveChoice=Total  F=50  SpecifyHarmonics=off  K=[0 1 2]  Ts=0
      settings: SourceProductBaseCode=PS
  RMS Measurement3 : eeRmsMeasurement/RMS Measurement  LabelModeActiveChoice=Total  F=50  SpecifyHarmonics=off  K=[0 1 2]  Ts=0
      settings: SourceProductBaseCode=PS
  Scope{6..10} (5 alike) : Scope
  input : PMIOPort  Side=Left
  input1 : PMIOPort  Port=2  Side=Left
  Q : Outport
  wires:
  Power Measurement2/2 -> Q/1
  PS-Simulink Converter3/1 -> RMS Measurement3/1, Scope8/1
  Power Measurement2/1 -> Display5/1, Scope10/1
  RMS Measurement2/1 -> Scope7/1, Display3/1, Power Measurement2/1
  PS-Simulink Converter2/1 -> RMS Measurement2/1, Scope6/1
  RMS Measurement3/1 -> Power Measurement2/2, Scope9/1, Display4/1
  connections:
  PS-Simulink Converter3/LConn1 -- input1/RConn1
  PS-Simulink Converter2/LConn1 -- input/RConn1

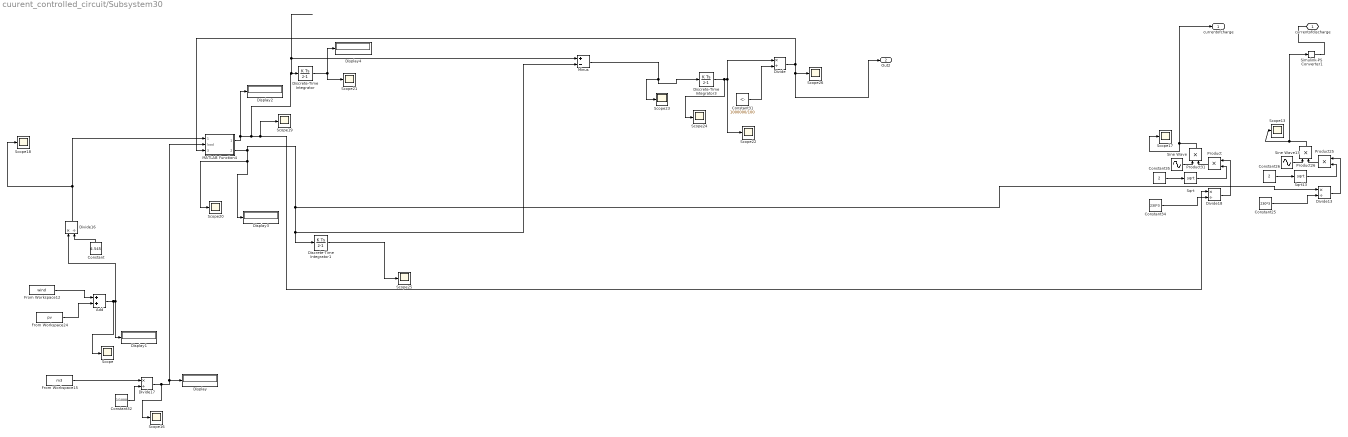
== system cuurent_controlled_circuit/Subsystem30 ==
  Add : Sum
  Constant : Constant  Value=4.545
  Constant25 : Constant  Value=230*3
  Constant26 : Constant  Value=2
  Constant31 : Constant  Value=1000000/100
  Constant32 : Constant  Value=1/1000
  Constant34 : Constant  Value=230*3
  Constant35 : Constant  Value=2
  Discrete-Time Integrator : DiscreteIntegrator  ICPrevOutput=DiscIntNeverNeededParam  ICPrevScaledInput=DiscIntNeverNeededParam
  Discrete-Time Integrator1 : DiscreteIntegrator  ICPrevOutput=DiscIntNeverNeededParam  ICPrevScaledInput=DiscIntNeverNeededParam
  Discrete-Time Integrator3 : DiscreteIntegrator  InitialCondition=500000  ICPrevOutput=DiscIntNeverNeededParam  ICPrevScaledInput=DiscIntNeverNeededParam
  Display{,1..4} (5 alike) : Display
  Divide{,13,16..18} (5 alike) : Product  Inputs=*/
  From Workspace12 : FromWorkspace  VariableName=wind  SampleTime=1  Interpolate=off  OutputAfterFinalValue=Holding final value
  From Workspace15 : FromWorkspace  VariableName=m3  SampleTime=1  Interpolate=off  OutputAfterFinalValue=Holding final value
  From Workspace24 : FromWorkspace  VariableName=pv  SampleTime=1  Interpolate=off  OutputAfterFinalValue=Holding final value
  MATLAB Function4 : MATLAB Function  TreatAsAtomicUnit=on
  Minus : Sum  Inputs=+-
  Product{,25..26,31} (4 alike) : Product
  Scope{,13,16..26} (13 alike) : Scope
  Simulink-PS Converter1 : nesl_utility/Simulink-PS Converter  PhysicalDomain=network_engine_domain  SubClassName=ps_input  LeftPortType=input  RightPortType=output  PseudoPeriodic=off  Frequencies=[]  NoiseDistribution=none  NoiseParameters=[]  Unit=1  AffineConversion=off  FilteringAndDerivatives=provide  SimscapeFilterOrder=1  InputFilterTimeConstant=0.001  UdotUserProvided=0
      settings: SourceProductBaseCode=SS,PW,VE
  Sine Wave : Sin  Frequency=314.6  SampleTime=0
  Sine Wave13 : Sin  Frequency=314.6  SampleTime=0
  Sqrt : Sqrt
  Sqrt13 : Sqrt
  currentofdischarge : PMIOPort  Side=Right
  currentofcharge : Outport
  Out2 : Outport  Port=2
  wires:
  MATLAB Function4/1(charge) -> Minus/1, Discrete-Time Integrator/1, Divide18/1, Scope19/1, Display2/1
  MATLAB Function4/2(discharge) -> Divide13/1, Minus/2, Discrete-Time Integrator1/1, Scope20/1, Display3/1
  Sine Wave13/1 -> Product26/1
  Product26/1 -> Simulink-PS Converter1/1, Scope13/1
  Discrete-Time Integrator/1 -> Display4/1, Scope21/1
  From Workspace24/1 -> Add/2
  Constant35/1 -> Sqrt/1
  Constant26/1 -> Sqrt13/1
  Product31/1 -> currentofcharge/1, Scope17/1
  Divide17/1 -> Scope16/1, MATLAB Function4/2(load), Display/1
  Divide13/1 -> Product25/1
  Add/1 -> Scope/1, Divide16/1, Display1/1
  Constant31/1 -> Divide/2
  Discrete-Time Integrator1/1 -> Scope25/1
  From Workspace15/1 -> Divide17/1
  Constant32/1 -> Divide17/2
  Minus/1 -> Discrete-Time Integrator3/1, Scope23/1
  Divide18/1 -> Product/1
  Discrete-Time Integrator3/1 -> Scope24/1, Divide/1, Scope22/1
  Product/1 -> Product31/2
  Product25/1 -> Product26/2
  Constant25/1 -> Divide13/2
  Constant/1 -> Divide16/2
  Divide16/1 -> Scope18/1, MATLAB Function4/1(pvandwind)
  Sine Wave/1 -> Product31/1
  Constant34/1 -> Divide18/2
  Sqrt/1 -> Product/2
  Sqrt13/1 -> Product25/2
  From Workspace12/1 -> Add/1
  Divide/1 -> Out2/1, Scope26/1, MATLAB Function4/3(batterycharge)
  connections:
  Simulink-PS Converter1/RConn1 -- currentofdischarge/RConn1

== system cuurent_controlled_circuit/Subsystem31 ==
  Add : Sum
  Constant : Constant  Value=4.545
  Constant25 : Constant  Value=230*3
  Constant26 : Constant  Value=2
  Constant31 : Constant  Value=1000000/100
  Constant32 : Constant  Value=1/1000
  Constant34 : Constant  Value=230*3
  Constant35 : Constant  Value=2
  Discrete-Time Integrator : DiscreteIntegrator  ICPrevOutput=DiscIntNeverNeededParam  ICPrevScaledInput=DiscIntNeverNeededParam
  Discrete-Time Integrator1 : DiscreteIntegrator  ICPrevOutput=DiscIntNeverNeededParam  ICPrevScaledInput=DiscIntNeverNeededParam
  Discrete-Time Integrator3 : DiscreteIntegrator  InitialCondition=500000  ICPrevOutput=DiscIntNeverNeededParam  ICPrevScaledInput=DiscIntNeverNeededParam
  Display{,1..4} (5 alike) : Display
  Divide{,13,16..18} (5 alike) : Product  Inputs=*/
  From Workspace12 : FromWorkspace  VariableName=wind  SampleTime=1  Interpolate=off  OutputAfterFinalValue=Holding final value
  From Workspace15 : FromWorkspace  VariableName=m3  SampleTime=1  Interpolate=off  OutputAfterFinalValue=Holding final value
  From Workspace24 : FromWorkspace  VariableName=pv  SampleTime=1  Interpolate=off  OutputAfterFinalValue=Holding final value
  MATLAB Function4 : MATLAB Function  TreatAsAtomicUnit=on
  Minus : Sum  Inputs=+-
  Product{,25..26,31} (4 alike) : Product
  Scope{,13,16..26} (13 alike) : Scope
  Simulink-PS Converter1 : nesl_utility/Simulink-PS Converter  PhysicalDomain=network_engine_domain  SubClassName=ps_input  LeftPortType=input  RightPortType=output  PseudoPeriodic=off  Frequencies=[]  NoiseDistribution=none  NoiseParameters=[]  Unit=1  AffineConversion=off  FilteringAndDerivatives=provide  SimscapeFilterOrder=1  InputFilterTimeConstant=0.001  UdotUserProvided=0
      settings: SourceProductBaseCode=SS,PW,VE
  Sine Wave : Sin  Frequency=314.6  Phase=120  SampleTime=0
  Sine Wave13 : Sin  Frequency=314.6  Phase=120  SampleTime=0
  Sqrt : Sqrt
  Sqrt13 : Sqrt
  currentofdischarge : PMIOPort  Side=Right
  currentofcharge : Outport
  wires:
  MATLAB Function4/1(charge) -> Minus/1, Discrete-Time Integrator/1, Divide18/1, Scope19/1, Display2/1
  MATLAB Function4/2(discharge) -> Divide13/1, Minus/2, Discrete-Time Integrator1/1, Scope20/1, Display3/1
  Divide/1 -> MATLAB Function4/3(batterycharge), Scope26/1
  Sine Wave13/1 -> Product26/1
  Product26/1 -> Simulink-PS Converter1/1, Scope13/1
  Discrete-Time Integrator/1 -> Display4/1, Scope21/1
  From Workspace24/1 -> Add/2
  Constant35/1 -> Sqrt/1
  Constant26/1 -> Sqrt13/1
  Product31/1 -> currentofcharge/1, Scope17/1
  Divide17/1 -> Scope16/1, MATLAB Function4/2(load), Display/1
  Divide13/1 -> Product25/1
  Add/1 -> Scope/1, Divide16/1, Display1/1
  Constant31/1 -> Divide/2
  Discrete-Time Integrator1/1 -> Scope25/1
  From Workspace15/1 -> Divide17/1
  Constant32/1 -> Divide17/2
  Minus/1 -> Discrete-Time Integrator3/1, Scope23/1
  Divide18/1 -> Product/1
  Discrete-Time Integrator3/1 -> Scope24/1, Divide/1, Scope22/1
  Product/1 -> Product31/2
  Product25/1 -> Product26/2
  Constant25/1 -> Divide13/2
  Constant/1 -> Divide16/2
  Divide16/1 -> Scope18/1, MATLAB Function4/1(pvandwind)
  Sine Wave/1 -> Product31/1
  Constant34/1 -> Divide18/2
  Sqrt/1 -> Product/2
  Sqrt13/1 -> Product25/2
  From Workspace12/1 -> Add/1
  connections:
  Simulink-PS Converter1/RConn1 -- currentofdischarge/RConn1

== system cuurent_controlled_circuit/Subsystem32 ==
  Add : Sum
  Constant : Constant  Value=4.545
  Constant25 : Constant  Value=230*3
  Constant26 : Constant  Value=2
  Constant31 : Constant  Value=1000000/100
  Constant32 : Constant  Value=1/1000
  Constant34 : Constant  Value=230*3
  Constant35 : Constant  Value=2
  Discrete-Time Integrator : DiscreteIntegrator  ICPrevOutput=DiscIntNeverNeededParam  ICPrevScaledInput=DiscIntNeverNeededParam
  Discrete-Time Integrator1 : DiscreteIntegrator  ICPrevOutput=DiscIntNeverNeededParam  ICPrevScaledInput=DiscIntNeverNeededParam
  Discrete-Time Integrator3 : DiscreteIntegrator  InitialCondition=500000  ICPrevOutput=DiscIntNeverNeededParam  ICPrevScaledInput=DiscIntNeverNeededParam
  Display{,1..4} (5 alike) : Display
  Divide{,13,16..18} (5 alike) : Product  Inputs=*/
  From Workspace12 : FromWorkspace  VariableName=wind  SampleTime=1  Interpolate=off  OutputAfterFinalValue=Holding final value
  From Workspace15 : FromWorkspace  VariableName=m3  SampleTime=1  Interpolate=off  OutputAfterFinalValue=Holding final value
  From Workspace24 : FromWorkspace  VariableName=pv  SampleTime=1  Interpolate=off  OutputAfterFinalValue=Holding final value
  MATLAB Function4 : MATLAB Function  TreatAsAtomicUnit=on
  Minus : Sum  Inputs=+-
  Product{,25..26,31} (4 alike) : Product
  Scope{,13,16..26} (13 alike) : Scope
  Simulink-PS Converter1 : nesl_utility/Simulink-PS Converter  PhysicalDomain=network_engine_domain  SubClassName=ps_input  LeftPortType=input  RightPortType=output  PseudoPeriodic=off  Frequencies=[]  NoiseDistribution=none  NoiseParameters=[]  Unit=1  AffineConversion=off  FilteringAndDerivatives=provide  SimscapeFilterOrder=1  InputFilterTimeConstant=0.001  UdotUserProvided=0
      settings: SourceProductBaseCode=SS,PW,VE
  Sine Wave : Sin  Frequency=314.6  Phase=240  SampleTime=0
  Sine Wave13 : Sin  Frequency=314.6  Phase=240  SampleTime=0
  Sqrt : Sqrt
  Sqrt13 : Sqrt
  currentofdischarge : PMIOPort  Side=Right
  currentofcharge : Outport
  wires:
  MATLAB Function4/1(charge) -> Minus/1, Discrete-Time Integrator/1, Divide18/1, Scope19/1, Display2/1
  MATLAB Function4/2(discharge) -> Divide13/1, Minus/2, Discrete-Time Integrator1/1, Scope20/1, Display3/1
  Divide/1 -> MATLAB Function4/3(batterycharge), Scope26/1
  Sine Wave13/1 -> Product26/1
  Product26/1 -> Simulink-PS Converter1/1, Scope13/1
  Discrete-Time Integrator/1 -> Display4/1, Scope21/1
  From Workspace24/1 -> Add/2
  Constant35/1 -> Sqrt/1
  Constant26/1 -> Sqrt13/1
  Product31/1 -> currentofcharge/1, Scope17/1
  Divide17/1 -> Scope16/1, MATLAB Function4/2(load), Display/1
  Divide13/1 -> Product25/1
  Add/1 -> Scope/1, Divide16/1, Display1/1
  Constant31/1 -> Divide/2
  Discrete-Time Integrator1/1 -> Scope25/1
  From Workspace15/1 -> Divide17/1
  Constant32/1 -> Divide17/2
  Minus/1 -> Discrete-Time Integrator3/1, Scope23/1
  Divide18/1 -> Product/1
  Discrete-Time Integrator3/1 -> Scope24/1, Divide/1, Scope22/1
  Product/1 -> Product31/2
  Product25/1 -> Product26/2
  Constant25/1 -> Divide13/2
  Constant/1 -> Divide16/2
  Divide16/1 -> Scope18/1, MATLAB Function4/1(pvandwind)
  Sine Wave/1 -> Product31/1
  Constant34/1 -> Divide18/2
  Sqrt/1 -> Product/2
  Sqrt13/1 -> Product25/2
  From Workspace12/1 -> Add/1
  connections:
  Simulink-PS Converter1/RConn1 -- currentofdischarge/RConn1

== system cuurent_controlled_circuit/Subsystem4 ==
  Display3 : Display
  Display4 : Display
  Display5 : Display
  PS-Simulink Converter2 : nesl_utility/PS-Simulink Converter  PhysicalDomain=network_engine_domain  SubClassName=ps_output  LeftPortType=input  RightPortType=output  PseudoPeriodic=off  Frequencies=[]  VectorFormat=inherit  Unit=inherit  AffineConversion=off
      settings: SourceProductBaseCode=SS,PW,VE
  PS-Simulink Converter3 : nesl_utility/PS-Simulink Converter  PhysicalDomain=network_engine_domain  SubClassName=ps_output  LeftPortType=input  RightPortType=output  PseudoPeriodic=off  Frequencies=[]  VectorFormat=inherit  Unit=inherit  AffineConversion=off
      settings: SourceProductBaseCode=SS,PW,VE
  Power Measurement2 : eePowerMeasurement/Power Measurement  LabelModeActiveChoice=Continuous  F=50  K=[0 1 2 3]  Ts=0
      settings: SourceProductBaseCode=PS
  RMS Measurement2 : eeRmsMeasurement/RMS Measurement  LabelModeActiveChoice=Total  F=50  SpecifyHarmonics=off  K=[0 1 2]  Ts=0
      settings: SourceProductBaseCode=PS
  RMS Measurement3 : eeRmsMeasurement/RMS Measurement  LabelModeActiveChoice=Total  F=50  SpecifyHarmonics=off  K=[0 1 2]  Ts=0
      settings: SourceProductBaseCode=PS
  Scope{6..10} (5 alike) : Scope
  input : PMIOPort  Side=Left
  input1 : PMIOPort  Port=2  Side=Left
  Q : Outport
  wires:
  Power Measurement2/2 -> Q/1
  PS-Simulink Converter3/1 -> RMS Measurement3/1, Scope8/1
  Power Measurement2/1 -> Display5/1, Scope10/1
  RMS Measurement2/1 -> Scope7/1, Display3/1, Power Measurement2/1
  PS-Simulink Converter2/1 -> RMS Measurement2/1, Scope6/1
  RMS Measurement3/1 -> Power Measurement2/2, Scope9/1, Display4/1
  connections:
  PS-Simulink Converter3/LConn1 -- input1/RConn1
  PS-Simulink Converter2/LConn1 -- input/RConn1
